simulink model "model_1"  (R2021b)
settings: Solver=VariableStepAuto  StartTime=0.0  StopTime=20  RelTol=1e-3
settings Model: Creator=vital  LastModifiedBy=kirba

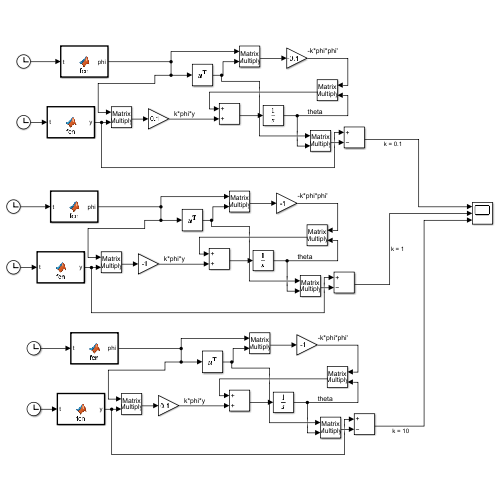
[thumbnail: Simulink's stored preview of the top-level diagram]
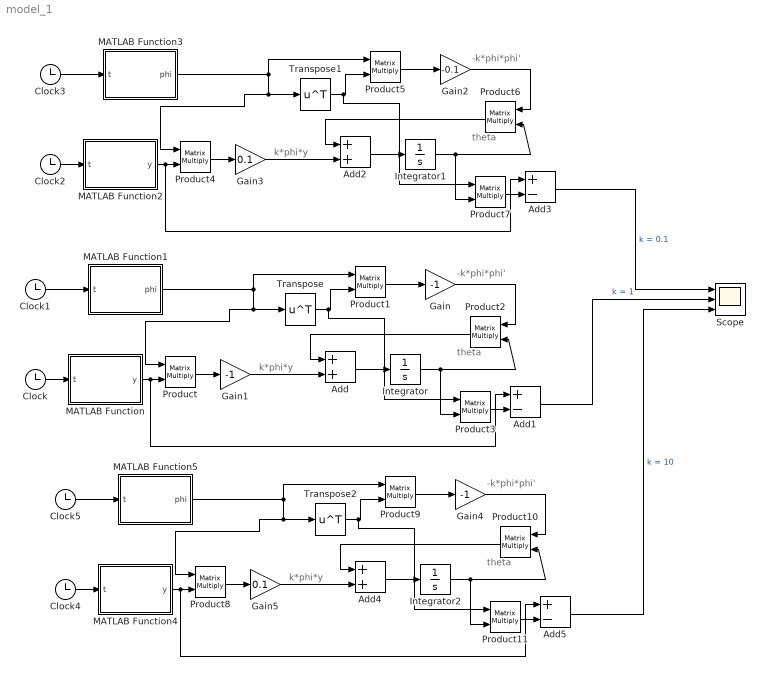
== system model_1 ==
  note: k*phi*y
  note: -k*phi*phi'
  note: theta
  note: -k*phi*phi'
  note: theta
  note: k*phi*y
  note: -k*phi*phi'
  note: theta
  note: k*phi*y
  Add : Sum
  Add1 : Sum  Inputs=+-
  Add2 : Sum
  Add3 : Sum  Inputs=+-
  Add4 : Sum
  Add5 : Sum  Inputs=+-
  Clock{,1..5} (6 alike) : Clock
  Gain : Gain  Gain=-1
  Gain1 : Gain  Gain=-1
  Gain2 : Gain  Gain=-0.1
  Gain3 : Gain  Gain=0.1
  Gain4 : Gain  Gain=-1
  Gain5 : Gain  Gain=0.1
  Integrator : Integrator
  Integrator1 : Integrator
  Integrator2 : Integrator
  MATLAB Function : MATLAB Function  TreatAsAtomicUnit=on
  MATLAB Function1 : MATLAB Function  TreatAsAtomicUnit=on
  MATLAB Function2 : MATLAB Function  TreatAsAtomicUnit=on
  MATLAB Function3 : MATLAB Function  TreatAsAtomicUnit=on
  MATLAB Function4 : MATLAB Function  TreatAsAtomicUnit=on
  MATLAB Function5 : MATLAB Function  TreatAsAtomicUnit=on
  Product{,1..11} (12 alike) : Product  Multiplication=Matrix(*)
  Scope : Scope  NumInputPorts=3
  Transpose : Math  Operator=transpose  SaturateOnIntegerOverflow=on
  Transpose1 : Math  Operator=transpose  SaturateOnIntegerOverflow=on
  Transpose2 : Math  Operator=transpose  SaturateOnIntegerOverflow=on
  wires:
  Clock1/1 -> MATLAB Function1/1(t)
  Transpose/1 -> Product3/1, Product1/2
  MATLAB Function1/1(phi) -> Product1/1, Product/1, Transpose/1
  Product1/1 -> Gain/1
  Clock/1 -> MATLAB Function/1(t)
  Gain/1 -> Product2/1
  Integrator/1 -> Product3/2, Product2/2
  Product2/1 -> Add/1
  MATLAB Function/1(y) -> Add1/1, Product/2
  Add/1 -> Integrator/1
  Product/1 -> Gain1/1
  Gain1/1 -> Add/2
  Product3/1 -> Add1/2
  Integrator1/1 -> Product7/2, Product6/2
  Gain3/1 -> Add2/2
  Product4/1 -> Gain3/1
  Product5/1 -> Gain2/1
  MATLAB Function2/1(y) -> Add3/1, Product4/2
  Product7/1 -> Add3/2
  Clock3/1 -> MATLAB Function3/1(t)
  Add2/1 -> Integrator1/1
  Transpose1/1 -> Product7/1, Product5/2
  Product6/1 -> Add2/1
  Gain2/1 -> Product6/1
  MATLAB Function3/1(phi) -> Product5/1, Product4/1, Transpose1/1
  Clock2/1 -> MATLAB Function2/1(t)
  Integrator2/1 -> Product11/2, Product10/2
  Gain5/1 -> Add4/2
  Product8/1 -> Gain5/1
  Product9/1 -> Gain4/1
  MATLAB Function4/1(y) -> Add5/1, Product8/2
  Product11/1 -> Add5/2
  Clock5/1 -> MATLAB Function5/1(t)
  Add4/1 -> Integrator2/1
  Transpose2/1 -> Product11/1, Product9/2
  Product10/1 -> Add4/1
  Gain4/1 -> Product10/1
  MATLAB Function5/1(phi) -> Product9/1, Product8/1, Transpose2/1
  Clock4/1 -> MATLAB Function4/1(t)
  Add5/1 -> Scope/3  "k = 10"
  Add1/1 -> Scope/2  "k = 1"
  Add3/1 -> Scope/1  "k = 0.1"

== matlab function model_1/MATLAB Function ==
  data: t input; y output
function y = fcn(t)

y = 5*cos(t+pi/3);

== matlab function model_1/MATLAB Function2 ==
  data: t input; y output
function y = fcn(t)

y = 5*cos(t+pi/3);

== matlab function model_1/MATLAB Function3 ==
  data: t input; phi output
function phi = fcn(t)

phi = [3*sin(t+pi/12); 5*cos(t + pi/8)];

== matlab function model_1/MATLAB Function4 ==
  data: t input; y output
function y = fcn(t)

y = 5*cos(t+pi/3);

== matlab function model_1/MATLAB Function5 ==
  data: t input; phi output
function phi = fcn(t)

phi = [3*sin(t+pi/12); 5*cos(t + pi/8)];

== matlab function model_1/MATLAB Function1 ==
  data: t input; phi output
function phi = fcn(t)

phi = [3*sin(t+pi/12); 5*cos(t + pi/8)];
